simulink model "reg_RST"  (Simulink 7.5)
settings: Solver=ode23s  StartTime=0.0  StopTime=3  FixedStep=T  RelTol=1e-3
values from neighbouring files (symbols this model uses):
  c = 75    [parametri.m]
  d = 0.05    [parametri.m]
  s = tf('s')    [parametri_RST.m]
  T = 1/w0    [parametri.m]    (also in parametri_RST.m)
  Tb = 1    [parametri.m]
  Tei = 2e-3    (= 0.002)    [parametri.m]
  Tm1 = 0.1    [parametri.m]
  Tm2 = 0.5    [parametri.m]
undefined symbols (not defined in the file or in its folder): p, q
settings Model: Creator=Tomislav  LastModifiedBy=Miha
settings OptimizationCC: InitFltsAndDblsToZero=on
settings DebuggingCC: StrictBusMsg=Warning

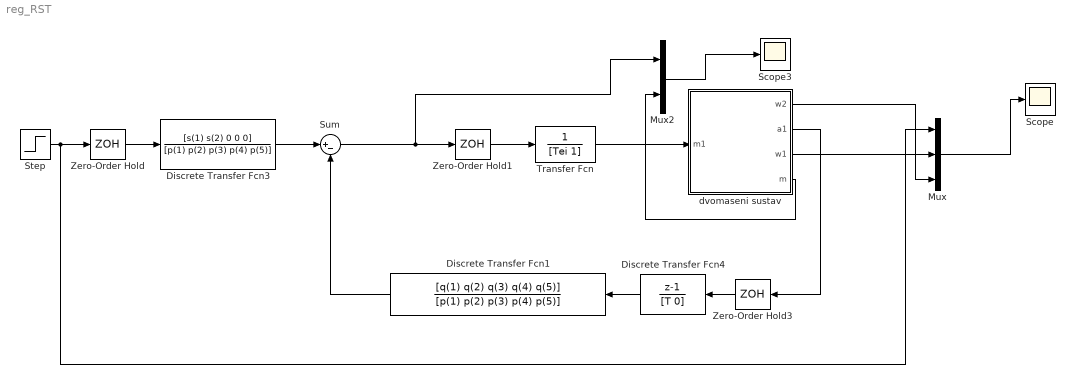
== system reg_RST ==
  Discrete Transfer Fcn1 : DiscreteTransferFcn  Numerator=[q(1) q(2) q(3) q(4) q(5)]  Denominator=[p(1) p(2) p(3) p(4) p(5)]  SampleTime=T
  Discrete Transfer Fcn3 : DiscreteTransferFcn  Numerator=[s(1) s(2) 0 0 0]  Denominator=[p(1) p(2) p(3) p(4) p(5)]  SampleTime=T
  Discrete Transfer Fcn4 : DiscreteTransferFcn  Numerator=[1 -1]  Denominator=[T 0]  SampleTime=T
  Mux : Mux  Inputs=3
  Mux2 : Mux  Inputs=2
  Scope : Scope
      settings: TimeRange=10  YMin=0.95  YMax=1.05  SaveName=w  DataFormat=Array
  Scope3 : Scope
      settings: TimeRange=10  YMin=-30000  YMax=10000  SaveName=m  DataFormat=Array
  Step : Step  Time=0  SampleTime=0
  Sum : Sum  Inputs=|+-  OutDataType=sfix(16)  OutScaling=2^0
  Transfer Fcn : TransferFcn  Denominator=[Tei 1]
  Zero-Order Hold : ZeroOrderHold  SampleTime=T
  Zero-Order Hold1 : ZeroOrderHold  SampleTime=T
  Zero-Order Hold3 : ZeroOrderHold  SampleTime=T
  dvomaseni sustav : Subsystem
  wires:
  Step/1 -> Zero-Order Hold/1, Mux/1
  Zero-Order Hold/1 -> Discrete Transfer Fcn3/1
  Zero-Order Hold1/1 -> Transfer Fcn/1
  Zero-Order Hold3/1 -> Discrete Transfer Fcn4/1
  Discrete Transfer Fcn4/1 -> Discrete Transfer Fcn1/1
  dvomaseni sustav/2(a1) -> Zero-Order Hold3/1
  dvomaseni sustav/3(w1) -> Mux/2
  Mux/1 -> Scope/1
  Mux2/1 -> Scope3/1
  dvomaseni sustav/4(m) -> Mux2/2
  Discrete Transfer Fcn1/1 -> Sum/2
  Sum/1 -> Zero-Order Hold1/1, Mux2/1
  Transfer Fcn/1 -> dvomaseni sustav/1(m1)
  Discrete Transfer Fcn3/1 -> Sum/1
  dvomaseni sustav/1(w2) -> Mux/3

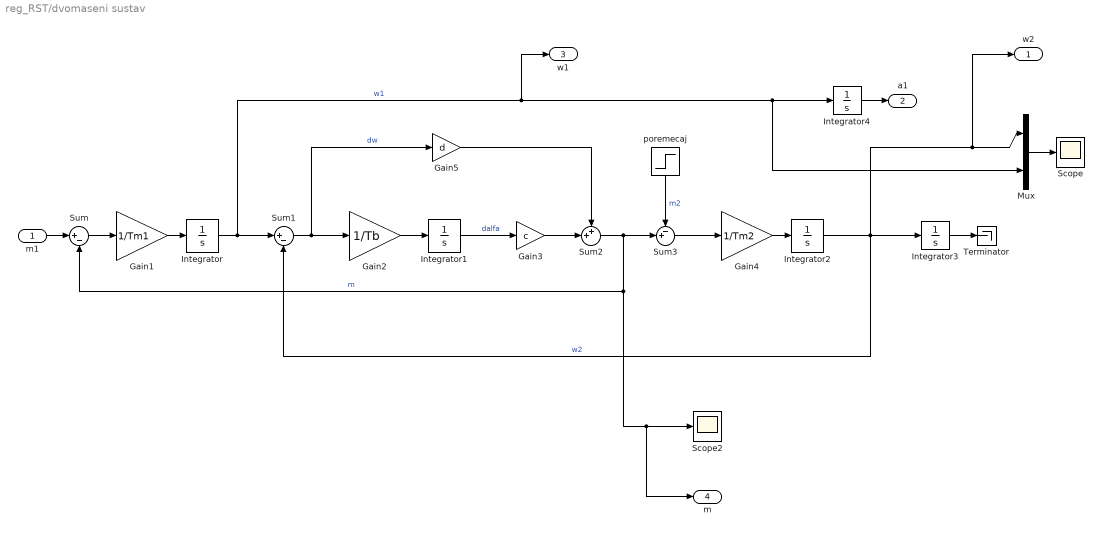
== system reg_RST/dvomaseni sustav ==
  m1 : Inport
  Gain1 : Gain  Gain=1/Tm1  ParameterDataType=sfix(16)  ParameterScaling=2^0  OutDataType=sfix(16)  OutScaling=2^0
  Gain2 : Gain  Gain=1/Tb  ParameterDataType=sfix(16)  ParameterScaling=2^0  OutDataType=sfix(16)  OutScaling=2^0
  Gain3 : Gain  Gain=c  ParameterDataType=sfix(16)  ParameterScaling=2^0  OutDataType=sfix(16)  OutScaling=2^0
  Gain4 : Gain  Gain=1/Tm2  ParameterDataType=sfix(16)  ParameterScaling=2^0  OutDataType=sfix(16)  OutScaling=2^0
  Gain5 : Gain  Gain=d  ParameterDataType=sfix(16)  ParameterScaling=2^0  OutDataType=sfix(16)  OutScaling=2^0
  Integrator{,1..4} (5 alike) : Integrator
  Mux : Mux  Inputs=2
  Scope : Scope
      settings: TimeRange=10  YMin=0  YMax=120
  Scope2 : Scope
      settings: TimeRange=10  YMin=-163622.0472440946  YMax=65669.29133858252  SaveName=m
  Sum : Sum  Inputs=|+-  OutDataType=sfix(16)  OutScaling=2^0
  Sum1 : Sum  Inputs=|+-  OutDataType=sfix(16)  OutScaling=2^0
  Sum2 : Sum  Inputs=++|  OutDataType=sfix(16)  OutScaling=2^0
  Sum3 : Sum  Inputs=-+|  OutDataType=sfix(16)  OutScaling=2^0
  Terminator : Terminator
  poremecaj : Step  Time=1.5  SampleTime=0
  w2 : Outport  OutDataType=sfix(16)  OutScaling=2^0
  a1 : Outport  Port=2  OutDataType=sfix(16)  OutScaling=2^0
  w1 : Outport  Port=3  OutDataType=fixdt(1, 16)  OutScaling=2^0
  m : Outport  Port=4  OutDataType=fixdt(1, 16)  OutScaling=2^0
  wires:
  Sum/1 -> Gain1/1
  Gain1/1 -> Integrator/1
  Integrator/1 -> Sum1/1, w1/1, Integrator4/1, Mux/2  "w1"
  Sum1/1 -> Gain2/1, Gain5/1  "dw"
  Gain2/1 -> Integrator1/1
  Integrator1/1 -> Gain3/1  "dalfa"
  Gain3/1 -> Sum2/2
  Sum2/1 -> Sum3/2, Sum/2, Scope2/1, m/1  "m"
  Gain4/1 -> Integrator2/1
  Integrator2/1 -> Sum1/2, Integrator3/1, Mux/1, w2/1  "w2"
  Sum3/1 -> Gain4/1
  Gain5/1 -> Sum2/1
  poremecaj/1 -> Sum3/1  "m2"
  m1/1 -> Sum/1
  Mux/1 -> Scope/1
  Integrator4/1 -> a1/1
  Integrator3/1 -> Terminator/1
